simulink model "ScpAp_SafetyStateManager"  (R2025b)
settings: Solver=FixedStepDiscrete  StartTime=0.0  StopTime=10.0  FixedStep=0.02  RelTol=1e-3
undefined symbols (not defined in the file or in its folder): VechSafetyStatus_L2p_IDT
settings Model: DataDictionary=EgasPOC.sldd  Creator=IAST283  LastModifiedBy=IAST283
settings DataIOCC: SaveFormat=StructureWithTime
settings OptimizationCC: DefaultParameterBehavior=Inlined  EnhancedBackFolding=on  PassReuseOutputArgsAs=Individual arguments  ZeroExternalMemoryAtStartup=off  ZeroInternalMemoryAtStartup=off  OptimizeBlockOrder=speed  DifferentSizesBufferReuse=on  OptimizationCustomize=off  EfficientTunableParamExpr=on
settings DebuggingCC: ParameterTunabilityLossMsg=error
settings SFSimCC: MATLABDynamicMemAlloc=off
settings RTWCC: SystemTargetFile=autosar.tlc  GenCodeOnly=on  TemplateMakefile=ert_default_tmf  DataTypeReplacement=CDataTypesFixedWidth  Description=AUTOSAR
settings CodeAppCC: ForceParamTrailComments=on  IgnoreCustomStorageClasses=off  OperatorAnnotations=on  SimulinkDataObjDesc=on  SFDataObjDesc=on  InsertBlockDesc=on
settings STFCustomTargetCC: SystemTargetFile=autosar.tlc  TargetLangStandard=C99 (ISO)  MultiwordLength=256.0  ParMdlRefBuildCompliant=on  CompOptLevelCompliant=on  ConcurrentExecutionCompliant=off  IncludeMdlTerminateFcn=off  CombineOutputUpdateFcns=on  SuppressErrorStatus=on  ERTCustomFileBanners=on  SupportNonFinite=off  SupportComplex=off  SupportContinuousTime=off  SupportNonInlinedSFcns=off  RemoveResetFunc=on  MATLABClassNameForMDSCustomization=Simulink.SoftwareTarget.ERTCustomization  AutosarCompliant=on  GRTInterface=off  UseToolchainInfoCompliant=on  LookupTableObjectStructAxisOrder=2,1,3,4,...  LUTObjectStructOrderEvenSpacing=Size,Table,Breakpoints  DisableAUTOSARRoutinesHostLibrary=off  AutosarSchemaVersion=R20-11  AutosarMaxShortNameLength=128.0  AutosarMatrixIOAsArray=off  AutosarCompilerAbstraction=off
settings ERTTargetCC: ERTCustomFileTemplate=example_file_process.tlc  BooleanTrueId=TRUE  BooleanFalseId=FALSE  TargetLangStandard=C99 (ISO)  ConcurrentExecutionCompliant=off  IncludeMdlTerminateFcn=off  SuppressErrorStatus=on  SupportNonFinite=off  SupportComplex=off  ModelStepFunctionPrototypeControlCompliant=off  CPPClassGenCompliant=off  AutosarCompliant=on  LookupTableObjectStructAxisOrder=2,1,3,4,...  LUTObjectStructOrderEvenSpacing=Size,Table,Breakpoints

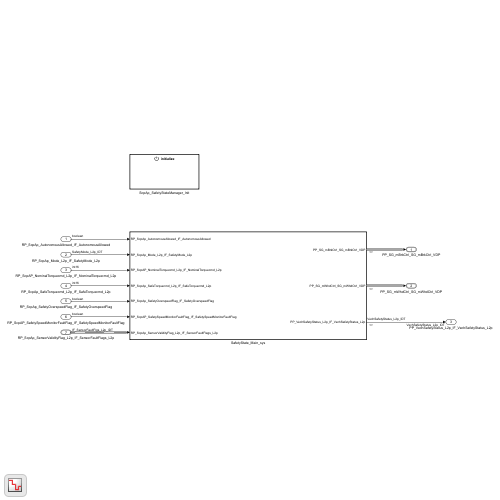
[thumbnail: Simulink's stored preview of the top-level diagram]
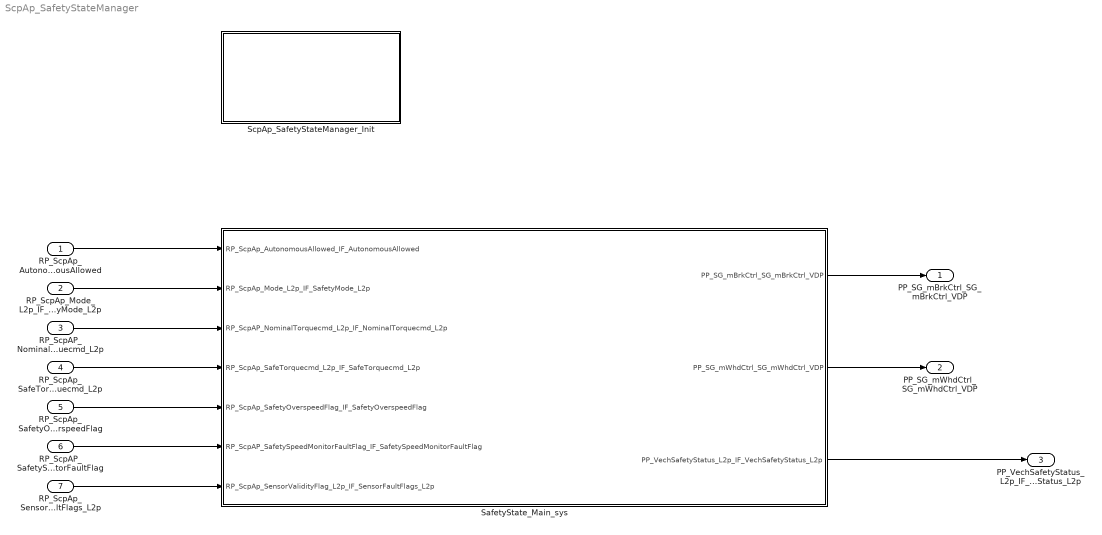
== system ScpAp_SafetyStateManager ==
  RP_ScpAp_AutonomousAllowed_IF_AutonomousAllowed : Inport  OutDataTypeStr=boolean  PortDimensions=1
  RP_ScpAp_Mode_L2p_IF_SafetyMode_L2p : Inport  Port=2  OutDataTypeStr=Enum: SafetyMode_L2p_IDT  PortDimensions=1
  RP_ScpAP_NominalTorquecmd_L2p_IF_NominalTorquecmd_L2p : Inport  Port=3  OutDataTypeStr=int16  PortDimensions=1
  RP_ScpAp_SafeTorquecmd_L2p_IF_SafeTorquecmd_L2p : Inport  Port=4  OutDataTypeStr=int16  PortDimensions=1
  RP_ScpAp_SafetyOverspeedFlag_IF_SafetyOverspeedFlag : Inport  Port=5  OutDataTypeStr=boolean  PortDimensions=1
  RP_ScpAP_SafetySpeedMonitorFaultFlag_IF_SafetySpeedMonitorFaultFlag : Inport  Port=6  OutDataTypeStr=boolean  PortDimensions=1
  RP_ScpAp_SensorValidityFlag_L2p_IF_SensorFaultFlags_L2p : Inport  Port=7  OutDataTypeStr=Bus: IF_SensorFaultFlgs_L2p_IDT  PortDimensions=1  BusOutputAsStruct=on
  SafetyState_Main_sys : Subsystem  TreatAsAtomicUnit=on  SystemSampleTime=0.02
  ScpAp_SafetyStateManager_Init : Subsystem
  PP_SG_mBrkCtrl_SG_mBrkCtrl_VDP : Outport  OutDataTypeStr=Bus: SG_mBrkCtrl_IDT  PortDimensions=1  BusOutputAsStruct=on
  PP_SG_mWhdCtrl_SG_mWhdCtrl_VDP : Outport  Port=2  OutDataTypeStr=Bus: SG_mWhdCtrl_IDT  PortDimensions=1  BusOutputAsStruct=on
  PP_VechSafetyStatus_L2p_IF_VechSafetyStatus_L2p : Outport  Port=3  OutDataTypeStr=Enum: VechSafetyStatus_L2p_IDT  PortDimensions=1
  wires:
  RP_ScpAp_AutonomousAllowed_IF_AutonomousAllowed/1 -> SafetyState_Main_sys/1(RP_ScpAp_AutonomousAllowed_IF_AutonomousAllowed)
  RP_ScpAp_Mode_L2p_IF_SafetyMode_L2p/1 -> SafetyState_Main_sys/2(RP_ScpAp_Mode_L2p_IF_SafetyMode_L2p)
  RP_ScpAP_NominalTorquecmd_L2p_IF_NominalTorquecmd_L2p/1 -> SafetyState_Main_sys/3(RP_ScpAP_NominalTorquecmd_L2p_IF_NominalTorquecmd_L2p)
  RP_ScpAp_SafeTorquecmd_L2p_IF_SafeTorquecmd_L2p/1 -> SafetyState_Main_sys/4(RP_ScpAp_SafeTorquecmd_L2p_IF_SafeTorquecmd_L2p)
  RP_ScpAp_SafetyOverspeedFlag_IF_SafetyOverspeedFlag/1 -> SafetyState_Main_sys/5(RP_ScpAp_SafetyOverspeedFlag_IF_SafetyOverspeedFlag)
  RP_ScpAP_SafetySpeedMonitorFaultFlag_IF_SafetySpeedMonitorFaultFlag/1 -> SafetyState_Main_sys/6(RP_ScpAP_SafetySpeedMonitorFaultFlag_IF_SafetySpeedMonitorFaultFlag)
  RP_ScpAp_SensorValidityFlag_L2p_IF_SensorFaultFlags_L2p/1 -> SafetyState_Main_sys/7(RP_ScpAp_SensorValidityFlag_L2p_IF_SensorFaultFlags_L2p)
  SafetyState_Main_sys/1(PP_SG_mBrkCtrl_SG_mBrkCtrl_VDP) -> PP_SG_mBrkCtrl_SG_mBrkCtrl_VDP/1
  SafetyState_Main_sys/2(PP_SG_mWhdCtrl_SG_mWhdCtrl_VDP) -> PP_SG_mWhdCtrl_SG_mWhdCtrl_VDP/1
  SafetyState_Main_sys/3(PP_VechSafetyStatus_L2p_IF_VechSafetyStatus_L2p) -> PP_VechSafetyStatus_L2p_IF_VechSafetyStatus_L2p/1

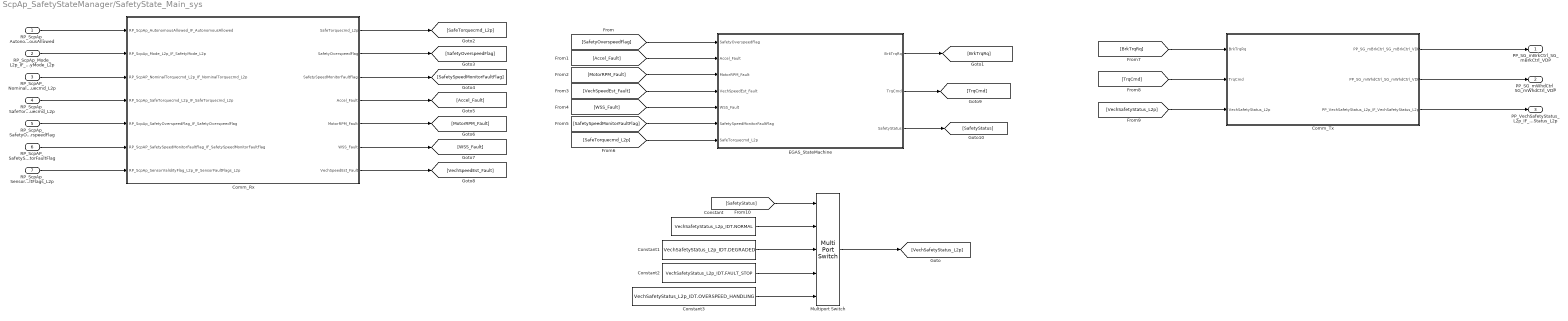
== system ScpAp_SafetyStateManager/SafetyState_Main_sys ==
  RP_ScpAp_AutonomousAllowed_IF_AutonomousAllowed : Inport
  RP_ScpAp_Mode_L2p_IF_SafetyMode_L2p : Inport  Port=2
  RP_ScpAP_NominalTorquecmd_L2p_IF_NominalTorquecmd_L2p : Inport  Port=3
  RP_ScpAp_SafeTorquecmd_L2p_IF_SafeTorquecmd_L2p : Inport  Port=4
  RP_ScpAp_SafetyOverspeedFlag_IF_SafetyOverspeedFlag : Inport  Port=5
  RP_ScpAP_SafetySpeedMonitorFaultFlag_IF_SafetySpeedMonitorFaultFlag : Inport  Port=6
  RP_ScpAp_SensorValidityFlag_L2p_IF_SensorFaultFlags_L2p : Inport  Port=7  OutDataTypeStr=Bus: IF_SensorFaultFlgs_L2p_IDT
  Comm_Rx : Subsystem  TreatAsAtomicUnit=on  SystemSampleTime=0.02
  Comm_Tx : Subsystem  TreatAsAtomicUnit=on  SystemSampleTime=0.02
  Constant : Constant  Value=VechSafetyStatus_L2p_IDT.NORMAL
  Constant1 : Constant  Value=VechSafetyStatus_L2p_IDT.DEGRADED
  Constant2 : Constant  Value=VechSafetyStatus_L2p_IDT.FAULT_STOP
  Constant3 : Constant  Value=VechSafetyStatus_L2p_IDT.OVERSPEED_HANDLING
  EGAS_StateMachine : Stateflow chart  TreatAsAtomicUnit=on  SystemSampleTime=0.02
  Multiport Switch : MultiPortSwitch  DataPortOrder=Zero-based contiguous  Inputs=4  zeroidx=on  SaturateOnIntegerOverflow=off  InputSameDT=off
  PP_SG_mBrkCtrl_SG_mBrkCtrl_VDP : Outport  OutDataTypeStr=Bus: SG_mBrkCtrl_IDT
  PP_SG_mWhdCtrl_SG_mWhdCtrl_VDP : Outport  Port=2  OutDataTypeStr=Bus: SG_mWhdCtrl_IDT
  PP_VechSafetyStatus_L2p_IF_VechSafetyStatus_L2p : Outport  Port=3  OutDataTypeStr=Enum: VechSafetyStatus_L2p_IDT
  wires:
  RP_ScpAp_AutonomousAllowed_IF_AutonomousAllowed/1 -> Comm_Rx/1(RP_ScpAp_AutonomousAllowed_IF_AutonomousAllowed)
  RP_ScpAp_Mode_L2p_IF_SafetyMode_L2p/1 -> Comm_Rx/2(RP_ScpAp_Mode_L2p_IF_SafetyMode_L2p)
  RP_ScpAP_NominalTorquecmd_L2p_IF_NominalTorquecmd_L2p/1 -> Comm_Rx/3(RP_ScpAP_NominalTorquecmd_L2p_IF_NominalTorquecmd_L2p)
  RP_ScpAp_SafeTorquecmd_L2p_IF_SafeTorquecmd_L2p/1 -> Comm_Rx/4(RP_ScpAp_SafeTorquecmd_L2p_IF_SafeTorquecmd_L2p)
  RP_ScpAp_SafetyOverspeedFlag_IF_SafetyOverspeedFlag/1 -> Comm_Rx/5(RP_ScpAp_SafetyOverspeedFlag_IF_SafetyOverspeedFlag)
  RP_ScpAP_SafetySpeedMonitorFaultFlag_IF_SafetySpeedMonitorFaultFlag/1 -> Comm_Rx/6(RP_ScpAP_SafetySpeedMonitorFaultFlag_IF_SafetySpeedMonitorFaultFlag)
  RP_ScpAp_SensorValidityFlag_L2p_IF_SensorFaultFlags_L2p/1 -> Comm_Rx/7(RP_ScpAp_SensorValidityFlag_L2p_IF_SensorFaultFlags_L2p)
  Comm_Rx/1(SafeTorquecmd_L2p) -> [SafeTorquecmd_L2p]
  Comm_Rx/2(SafetyOverspeedFlag) -> [SafetyOverspeedFlag]
  Comm_Rx/3(SafetySpeedMonitorFaultFlag) -> [SafetySpeedMonitorFaultFlag]
  Comm_Rx/4(Accel_Fault) -> [Accel_Fault]
  Comm_Rx/5(MotorRPM_Fault) -> [MotorRPM_Fault]
  Comm_Rx/6(WSS_Fault) -> [WSS_Fault]
  Comm_Rx/7(VechSpeedEst_Fault) -> [VechSpeedEst_Fault]
  [SafetyOverspeedFlag] -> EGAS_StateMachine/1(SafetyOverspeedFlag)
  [Accel_Fault] -> EGAS_StateMachine/2(Accel_Fault)
  [MotorRPM_Fault] -> EGAS_StateMachine/3(MotorRPM_Fault)
  [VechSpeedEst_Fault] -> EGAS_StateMachine/4(VechSpeedEst_Fault)
  [WSS_Fault] -> EGAS_StateMachine/5(WSS_Fault)
  [SafetySpeedMonitorFaultFlag] -> EGAS_StateMachine/6(SafetySpeedMonitorFaultFlag)
  [SafeTorquecmd_L2p] -> EGAS_StateMachine/7(SafeTorquecmd_L2p)
  EGAS_StateMachine/1(BrkTrqRq) -> [BrkTrqRq]
  EGAS_StateMachine/2(TrqCmd) -> [TrqCmd]
  Comm_Tx/1(PP_SG_mBrkCtrl_SG_mBrkCtrl_VDP) -> PP_SG_mBrkCtrl_SG_mBrkCtrl_VDP/1
  Comm_Tx/2(PP_SG_mWhdCtrl_SG_mWhdCtrl_VDP) -> PP_SG_mWhdCtrl_SG_mWhdCtrl_VDP/1
  Comm_Tx/3(PP_VechSafetyStatus_L2p_IF_VechSafetyStatus_L2p) -> PP_VechSafetyStatus_L2p_IF_VechSafetyStatus_L2p/1
  [BrkTrqRq] -> Comm_Tx/1(BrkTrqRq)
  [TrqCmd] -> Comm_Tx/2(TrqCmd)
  [VechSafetyStatus_L2p] -> Comm_Tx/3(VechSafetyStatus_L2p)
  EGAS_StateMachine/3(SafetyStatus) -> [SafetyStatus]
  Multiport Switch/1 -> [VechSafetyStatus_L2p]
  [SafetyStatus] -> Multiport Switch/1
  Constant/1 -> Multiport Switch/2
  Constant1/1 -> Multiport Switch/3
  Constant2/1 -> Multiport Switch/4
  Constant3/1 -> Multiport Switch/5

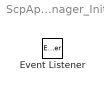
== system ScpAp_SafetyStateManager/ScpAp_SafetyStateManager_Init ==
  Event Listener : EventListener  EventName=reset

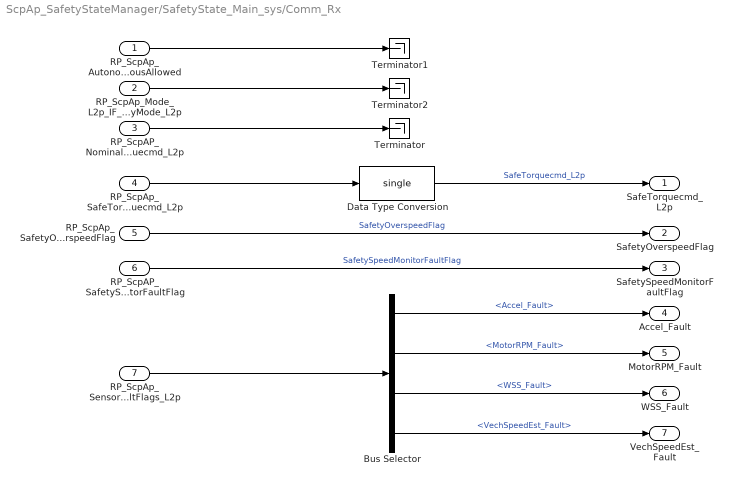
== system ScpAp_SafetyStateManager/SafetyState_Main_sys/Comm_Rx ==
  RP_ScpAp_AutonomousAllowed_IF_AutonomousAllowed : Inport
  RP_ScpAp_Mode_L2p_IF_SafetyMode_L2p : Inport  Port=2
  RP_ScpAP_NominalTorquecmd_L2p_IF_NominalTorquecmd_L2p : Inport  Port=3
  RP_ScpAp_SafeTorquecmd_L2p_IF_SafeTorquecmd_L2p : Inport  Port=4
  RP_ScpAp_SafetyOverspeedFlag_IF_SafetyOverspeedFlag : Inport  Port=5
  RP_ScpAP_SafetySpeedMonitorFaultFlag_IF_SafetySpeedMonitorFaultFlag : Inport  Port=6
  RP_ScpAp_SensorValidityFlag_L2p_IF_SensorFaultFlags_L2p : Inport  Port=7  OutDataTypeStr=Bus: IF_SensorFaultFlgs_L2p_IDT
  Bus Selector : BusSelector  OutputSignals=Accel_Fault,MotorRPM_Fault,WSS_Fault,VechSpeedEst_Fault
  Data Type Conversion : DataTypeConversion  OutDataTypeStr=single  SaturateOnIntegerOverflow=off  RndMeth=Floor
  Terminator : Terminator
  Terminator1 : Terminator
  Terminator2 : Terminator
  SafeTorquecmd_L2p : Outport
  SafetyOverspeedFlag : Outport  Port=2
  SafetySpeedMonitorFaultFlag : Outport  Port=3
  Accel_Fault : Outport  Port=4
  MotorRPM_Fault : Outport  Port=5
  WSS_Fault : Outport  Port=6
  VechSpeedEst_Fault : Outport  Port=7
  wires:
  RP_ScpAP_NominalTorquecmd_L2p_IF_NominalTorquecmd_L2p/1 -> Terminator/1
  Bus Selector/3 -> WSS_Fault/1  "<WSS_Fault>"
  Bus Selector/1 -> Accel_Fault/1  "<Accel_Fault>"
  Bus Selector/2 -> MotorRPM_Fault/1  "<MotorRPM_Fault>"
  Bus Selector/4 -> VechSpeedEst_Fault/1  "<VechSpeedEst_Fault>"
  RP_ScpAP_SafetySpeedMonitorFaultFlag_IF_SafetySpeedMonitorFaultFlag/1 -> SafetySpeedMonitorFaultFlag/1  "SafetySpeedMonitorFaultFlag"
  RP_ScpAp_SafetyOverspeedFlag_IF_SafetyOverspeedFlag/1 -> SafetyOverspeedFlag/1  "SafetyOverspeedFlag"
  RP_ScpAp_SafeTorquecmd_L2p_IF_SafeTorquecmd_L2p/1 -> Data Type Conversion/1
  RP_ScpAp_SensorValidityFlag_L2p_IF_SensorFaultFlags_L2p/1 -> Bus Selector/1
  RP_ScpAp_AutonomousAllowed_IF_AutonomousAllowed/1 -> Terminator1/1
  RP_ScpAp_Mode_L2p_IF_SafetyMode_L2p/1 -> Terminator2/1
  Data Type Conversion/1 -> SafeTorquecmd_L2p/1  "SafeTorquecmd_L2p"

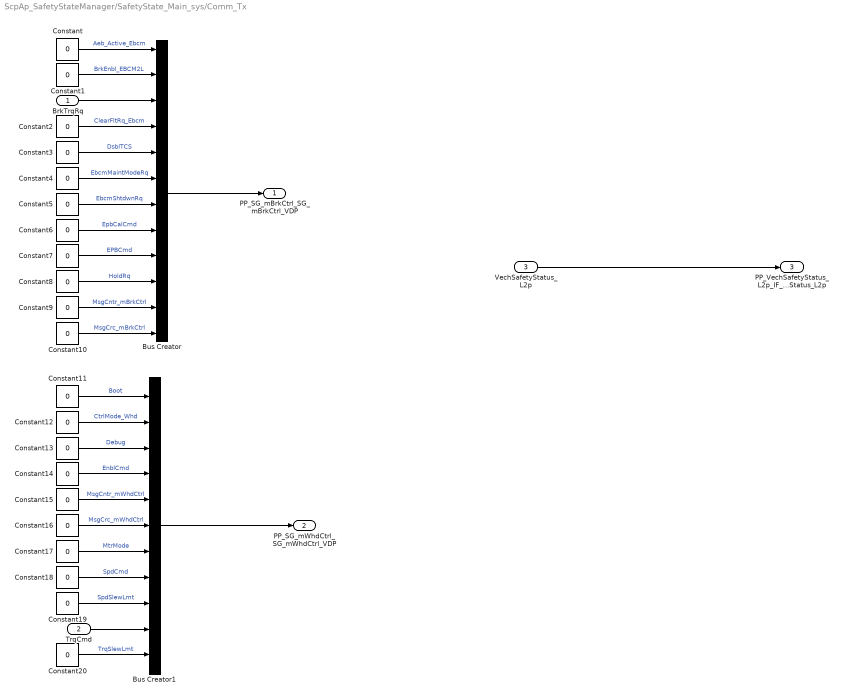
== system ScpAp_SafetyStateManager/SafetyState_Main_sys/Comm_Tx ==
  BrkTrqRq : Inport
  TrqCmd : Inport  Port=2
  VechSafetyStatus_L2p : Inport  Port=3  OutDataTypeStr=Enum: VechSafetyStatus_L2p_IDT
  Bus Creator : BusCreator  Inputs=12  OutDataTypeStr=Bus: SG_mBrkCtrl_IDT
  Bus Creator1 : BusCreator  Inputs=11  OutDataTypeStr=Bus: SG_mWhdCtrl_IDT
  Constant{,1..6,8,11,13..14} (11 alike) : Constant  Value=0  OutDataTypeStr=boolean
  Constant{7,9..10,12,15..17} (7 alike) : Constant  Value=0  OutDataTypeStr=uint8
  Constant18 : Constant  Value=0  OutDataTypeStr=single
  Constant19 : Constant  Value=0  OutDataTypeStr=single
  Constant20 : Constant  Value=0  OutDataTypeStr=single
  PP_SG_mBrkCtrl_SG_mBrkCtrl_VDP : Outport  OutDataTypeStr=Bus: SG_mBrkCtrl_IDT
  PP_SG_mWhdCtrl_SG_mWhdCtrl_VDP : Outport  Port=2  OutDataTypeStr=Bus: SG_mWhdCtrl_IDT
  PP_VechSafetyStatus_L2p_IF_VechSafetyStatus_L2p : Outport  Port=3  OutDataTypeStr=Enum: VechSafetyStatus_L2p_IDT
  wires:
  VechSafetyStatus_L2p/1 -> PP_VechSafetyStatus_L2p_IF_VechSafetyStatus_L2p/1
  Bus Creator/1 -> PP_SG_mBrkCtrl_SG_mBrkCtrl_VDP/1
  Bus Creator1/1 -> PP_SG_mWhdCtrl_SG_mWhdCtrl_VDP/1
  BrkTrqRq/1 -> Bus Creator/3
  Constant/1 -> Bus Creator/1  "Aeb_Active_Ebcm"
  Constant1/1 -> Bus Creator/2  "BrkEnbl_EBCM2L"
  Constant2/1 -> Bus Creator/4  "ClearFltRq_Ebcm"
  Constant3/1 -> Bus Creator/5  "DsblTCS"
  Constant4/1 -> Bus Creator/6  "EbcmMaintModeRq"
  Constant5/1 -> Bus Creator/7  "EbcmShtdwnRq"
  Constant6/1 -> Bus Creator/8  "EpbCalCmd"
  Constant7/1 -> Bus Creator/9  "EPBCmd"
  Constant8/1 -> Bus Creator/10  "HoldRq"
  Constant9/1 -> Bus Creator/11  "MsgCntr_mBrkCtrl"
  Constant10/1 -> Bus Creator/12  "MsgCrc_mBrkCtrl"
  TrqCmd/1 -> Bus Creator1/10
  Constant11/1 -> Bus Creator1/1  "Boot"
  Constant12/1 -> Bus Creator1/2  "CtrlMode_Whd"
  Constant20/1 -> Bus Creator1/11  "TrqSlewLmt"
  Constant19/1 -> Bus Creator1/9  "SpdSlewLmt"
  Constant18/1 -> Bus Creator1/8  "SpdCmd"
  Constant17/1 -> Bus Creator1/7  "MtrMode"
  Constant16/1 -> Bus Creator1/6  "MsgCrc_mWhdCtrl"
  Constant13/1 -> Bus Creator1/3  "Debug"
  Constant14/1 -> Bus Creator1/4  "EnblCmd"
  Constant15/1 -> Bus Creator1/5  "MsgCntr_mWhdCtrl"

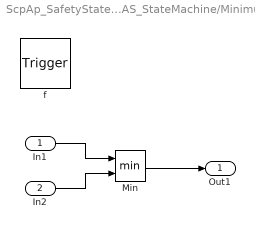
== system ScpAp_SafetyStateManager/SafetyState_Main_sys/EGAS_StateMachine/Minimum ==
  In1 : Inport  OutDataTypeStr=single  PortDimensions=1
  In2 : Inport  Port=2  OutDataTypeStr=single  PortDimensions=1
  f : TriggerPort  TriggerType=function-call  VariantControl=(inherit)
      settings: CopyFcn=Stateflow.SLINSF.SimulinkMan.removeBlockPreDeleteFcn  PreDeleteFcn=Stateflow.SLINSF.SimulinkMan.unsafePredeleteFcn
  Min : MinMax  Inputs=2
  Out1 : Outport
  wires:
  In1/1 -> Min/1
  In2/1 -> Min/2
  Min/1 -> Out1/1

== stateflow chart ScpAp_SafetyStateManager/SafetyState_Main_sys/EGAS_StateMachine ==
  state Normal
    en:
    SafetyStatus=0;
    BrkTrqRq=0;
    TrqCmd=SafeTorquecmd_L2p;
    du:
    SafetyStatus=0;
    BrkTrqRq=0;
    TrqCmd=SafeTorquecmd_L2p;
  state OverSpeed_Handling
    en:
    TrqCmd=Minimum(SafeTorquecmd_L2p,Torque_Decel_Limit);
    BrkTrqRq=Brake_Decel_Level;
    SafetyStatus=3;
    du:
    TrqCmd=Minimum(SafeTorquecmd_L2p,Torque_Decel_Limit);
    BrkTrqRq=Brake_Decel_Level;
    SafetyStatus=3;
  state Out1 = Minimum(In1,In2) [function]
  state Degrade
    en:
    TrqCmd=0;
    BrkTrqRq=Brake_Limp;
    SafetyStatus=1;
    du:
    TrqCmd=0;
    BrkTrqRq=Brake_Limp;
    SafetyStatus=1;
  state Energency_Stop
    en:
    TrqCmd=0;
    BrkTrqRq=Brake_Max_Safe;
    SafetyStatus=2;
    du:
    TrqCmd=0;
    BrkTrqRq=Brake_Max_Safe;
    SafetyStatus=2;
  (default) -> Normal
  Normal -> OverSpeed_Handling [order 1] : [SafetyOverspeedFlag == 1]
  OverSpeed_Handling -> Normal [order 1] : [[SafetyOverspeedFlag == 0 && Accel_Fault == 0 && MotorRPM_Fault == 0 && WSS_Fault == 0 && VechSpeedEst_Fault == 0]]
  Degrade -> Normal [order 2] : [SafetySpeedMonitorFaultFlag == 0 && SafetyOverspeedFlag == 0 && Accel_Fault == 0 && MotorRPM_Fault == 0 && WSS_Fault == 0 && VechSpeedEst_Fault == 0]
  Normal -> Degrade [order 2] : [SafetySpeedMonitorFaultFlag == 1 || Accel_Fault == 1 && MotorRPM_Fault == 1 && WSS_Fault == 1 && VechSpeedEst_Fault == 1]
  OverSpeed_Handling -> Degrade [order 2] : [[SafetySpeedMonitorFaultFlag == 1 || Accel_Fault == 1 && MotorRPM_Fault == 1 && WSS_Fault == 1 && VechSpeedEst_Fault == 1]]
  Degrade -> Energency_Stop [order 1] : [after(60, msec)]
  data: In1 function_input single size=1; In2 function_input single size=1; Out1 function_output; SafetyOverspeedFlag input; Accel_Fault input; MotorRPM_Fault input; VechSpeedEst_Fault input; WSS_Fault input; SafetySpeedMonitorFaultFlag input; BrkTrqRq output single; TrqCmd output single; SafeTorquecmd_L2p input; Brake_Decel_Level local single =500; Brake_Limp local single =600; Brake_Max_Safe local single =800; Torque_Decel_Limit local single =500; SafetyStatus output int8
